simulink model "Simulation_Suspension_System"  (R2020b)
settings: Solver=ode4  StartTime=0.0  StopTime=10.0  FixedStep=0.01  RelTol=1e-3
InitFcn:
  | M=900;
  | m=40;
  | I=1506.645875;
  | k1=14.64*3500;
  | k2=14.64*3500;
  | k3=91.5*3000;
  | k4=91.5*3000;
  | c1=64.05*40;
  | c2=64.05*40;
  | c3=2748.66*3;
  | c4=2748.66*3;
  | a=2.635;
  | b=1.3;
settings Model: Creator=Amir  LastModifiedBy=vahed
settings DataIOCC: ReturnWorkspaceOutputs=off
settings DebuggingCC: ArithmeticOperatorsInVariantConditions=warning
settings SFSimCC: CustomCodeUndefinedFunction=UseInterfaceOnly

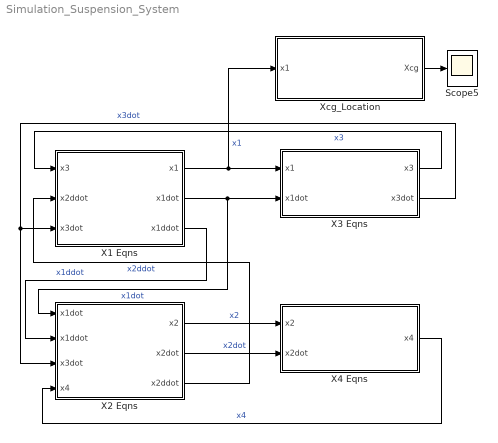
== system Simulation_Suspension_System ==
  Scope5 : Scope
  X1 Eqns : Subsystem
  X2 Eqns : Subsystem
  X3 Eqns : Subsystem
  X4 Eqns : Subsystem
  Xcg_Location : Subsystem
  wires:
  X3 Eqns/2(x3dot) -> X2 Eqns/3(x3dot), X1 Eqns/3(x3dot)  "x3dot"
  Xcg_Location/1(Xcg) -> Scope5/1
  X4 Eqns/1(x4) -> X2 Eqns/4(x4)  "x4"
  X2 Eqns/2(x2dot) -> X4 Eqns/2(x2dot)  "x2dot"
  X2 Eqns/1(x2) -> X4 Eqns/1(x2)  "x2"
  X1 Eqns/2(x1dot) -> X2 Eqns/1(x1dot), X3 Eqns/2(x1dot)  "x1dot"
  X1 Eqns/1(x1) -> X3 Eqns/1(x1), Xcg_Location/1(x1)  "x1"
  X2 Eqns/3(x2ddot) -> X1 Eqns/2(x2ddot)  "x2ddot"
  X3 Eqns/1(x3) -> X1 Eqns/1(x3)  "x3"
  X1 Eqns/3(x1ddot) -> X2 Eqns/2(x1ddot)  "x1ddot"

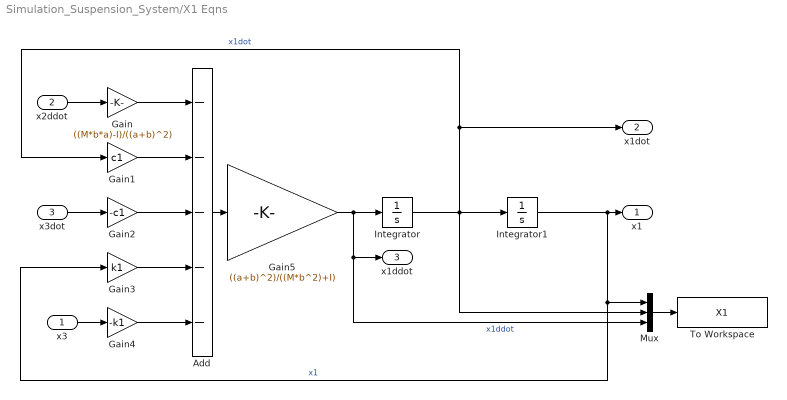
== system Simulation_Suspension_System/X1 Eqns ==
  x3 : Inport
  x2ddot : Inport  Port=2
  x3dot : Inport  Port=3
  Add : Sum  Inputs=-----
  Gain : Gain  Gain=((M*b*a)-I)/((a+b)^2)
  Gain1 : Gain  Gain=c1
  Gain2 : Gain  Gain=-c1
  Gain3 : Gain  Gain=k1
  Gain4 : Gain  Gain=-k1
  Gain5 : Gain  Gain=((a+b)^2)/((M*b^2)+I)
  Integrator : Integrator
  Integrator1 : Integrator  InitialCondition=0.2
  Mux : Mux  Inputs=3
  To Workspace : ToWorkspace  VariableName=X1  SaveFormat=Timeseries  SampleTime=-1
  x1 : Outport
  x1dot : Outport  Port=2
  x1ddot : Outport  Port=3
  wires:
  Add/1 -> Gain5/1
  Gain2/1 -> Add/3
  Gain/1 -> Add/1
  Integrator/1 -> Mux/2, Gain1/1, x1dot/1, Integrator1/1  "x1dot"
  Gain5/1 -> Mux/3, x1ddot/1, Integrator/1  "x1ddot"
  Gain1/1 -> Add/2
  Gain4/1 -> Add/5
  Gain3/1 -> Add/4
  x2ddot/1 -> Gain/1
  x3/1 -> Gain4/1
  x3dot/1 -> Gain2/1
  Integrator1/1 -> Mux/1, Gain3/1, x1/1  "x1"
  Mux/1 -> To Workspace/1

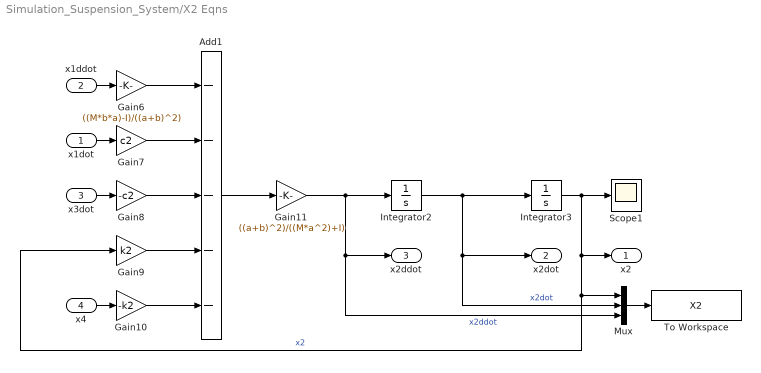
== system Simulation_Suspension_System/X2 Eqns ==
  x1dot : Inport
  x1ddot : Inport  Port=2
  x3dot : Inport  Port=3
  x4 : Inport  Port=4
  Add1 : Sum  Inputs=-----
  Gain10 : Gain  Gain=-k2
  Gain11 : Gain  Gain=((a+b)^2)/((M*a^2)+I)
  Gain6 : Gain  Gain=((M*b*a)-I)/((a+b)^2)
  Gain7 : Gain  Gain=c2
  Gain8 : Gain  Gain=-c2
  Gain9 : Gain  Gain=k2
  Integrator2 : Integrator
  Integrator3 : Integrator  InitialCondition=-0.15
  Mux : Mux  Inputs=3
  Scope1 : Scope
  To Workspace : ToWorkspace  VariableName=X2  SaveFormat=Timeseries  SampleTime=-1
  x2 : Outport
  x2dot : Outport  Port=2
  x2ddot : Outport  Port=3
  wires:
  x3dot/1 -> Gain8/1
  Gain11/1 -> Mux/3, x2ddot/1, Integrator2/1  "x2ddot"
  Integrator3/1 -> Mux/1, Gain9/1, x2/1, Scope1/1  "x2"
  Add1/1 -> Gain11/1
  Gain8/1 -> Add1/3
  Gain7/1 -> Add1/2
  Integrator2/1 -> Mux/2, x2dot/1, Integrator3/1  "x2dot"
  Gain6/1 -> Add1/1
  Gain9/1 -> Add1/4
  Gain10/1 -> Add1/5
  x4/1 -> Gain10/1
  x1ddot/1 -> Gain6/1
  x1dot/1 -> Gain7/1
  Mux/1 -> To Workspace/1

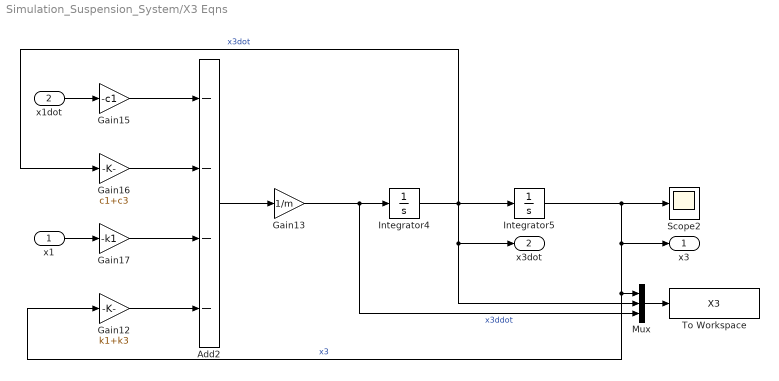
== system Simulation_Suspension_System/X3 Eqns ==
  x1 : Inport
  x1dot : Inport  Port=2
  Add2 : Sum  Inputs=----
  Gain12 : Gain  Gain=k1+k3
  Gain13 : Gain  Gain=1/m
  Gain15 : Gain  Gain=-c1
  Gain16 : Gain  Gain=c1+c3
  Gain17 : Gain  Gain=-k1
  Integrator4 : Integrator
  Integrator5 : Integrator
  Mux : Mux  Inputs=3
  Scope2 : Scope
  To Workspace : ToWorkspace  VariableName=X3  SaveFormat=Timeseries  SampleTime=-1
  x3 : Outport
  x3dot : Outport  Port=2
  wires:
  Gain13/1 -> Mux/3, Integrator4/1  "x3ddot"
  Add2/1 -> Gain13/1
  Gain16/1 -> Add2/2
  Integrator4/1 -> Mux/2, x3dot/1, Gain16/1, Integrator5/1  "x3dot"
  Integrator5/1 -> Scope2/1, Mux/1, Gain12/1, x3/1  "x3"
  Gain15/1 -> Add2/1
  Gain17/1 -> Add2/3
  Gain12/1 -> Add2/4
  x1dot/1 -> Gain15/1
  x1/1 -> Gain17/1
  Mux/1 -> To Workspace/1

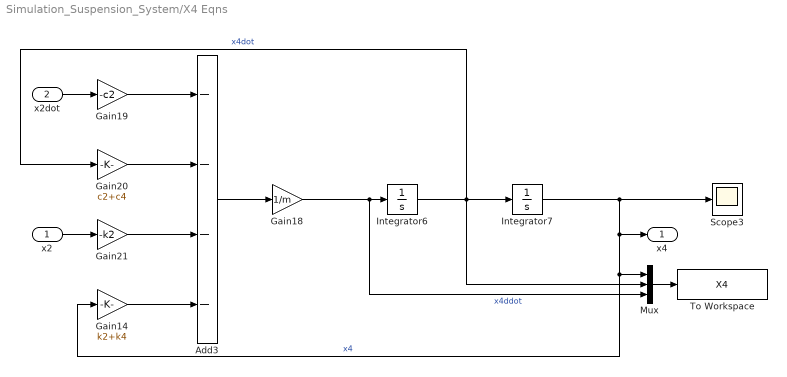
== system Simulation_Suspension_System/X4 Eqns ==
  x2 : Inport
  x2dot : Inport  Port=2
  Add3 : Sum  Inputs=----
  Gain14 : Gain  Gain=k2+k4
  Gain18 : Gain  Gain=1/m
  Gain19 : Gain  Gain=-c2
  Gain20 : Gain  Gain=c2+c4
  Gain21 : Gain  Gain=-k2
  Integrator6 : Integrator
  Integrator7 : Integrator
  Mux : Mux  Inputs=3
  Scope3 : Scope
  To Workspace : ToWorkspace  VariableName=X4  SaveFormat=Timeseries  SampleTime=-1
  x4 : Outport
  wires:
  Gain14/1 -> Add3/4
  Integrator7/1 -> Scope3/1, Mux/1, Gain14/1, x4/1  "x4"
  Gain21/1 -> Add3/3
  Gain19/1 -> Add3/1
  Integrator6/1 -> Mux/2, Gain20/1, Integrator7/1  "x4dot"
  Gain18/1 -> Mux/3, Integrator6/1  "x4ddot"
  Add3/1 -> Gain18/1
  Gain20/1 -> Add3/2
  x2dot/1 -> Gain19/1
  x2/1 -> Gain21/1
  Mux/1 -> To Workspace/1

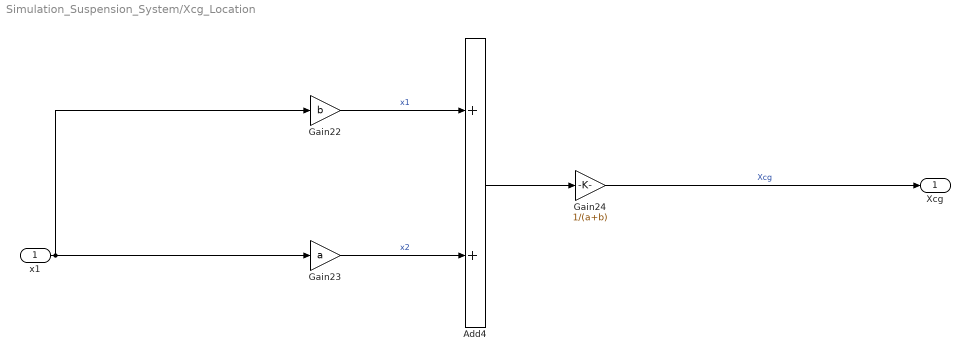
== system Simulation_Suspension_System/Xcg_Location ==
  x1 : Inport
  Add4 : Sum
  Gain22 : Gain  Gain=b
  Gain23 : Gain  Gain=a
  Gain24 : Gain  Gain=1/(a+b)
  Xcg : Outport
  wires:
  Gain24/1 -> Xcg/1  "Xcg"
  Gain23/1 -> Add4/2  "x2"
  x1/1 -> Gain22/1, Gain23/1
  Gain22/1 -> Add4/1  "x1"
  Add4/1 -> Gain24/1
